simulink model "Lab_Electrical_System"  (R2018a)
settings: Solver=VariableStepAuto  StartTime=0.0  StopTime=10  RelTol=1e-3
libraries: dspsrcs4 x1
settings Model: Creator=samak-twins  LastModifiedBy=samak

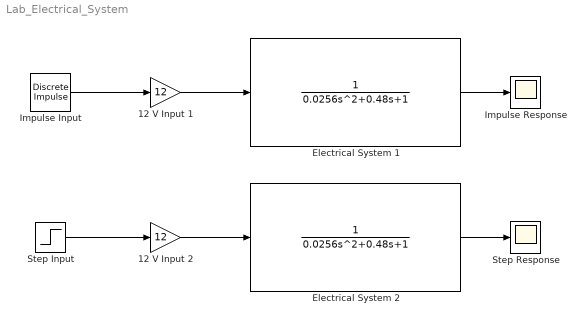
== system Lab_Electrical_System ==
  12 V Input 1 : Gain  Gain=12
  12 V Input 2 : Gain  Gain=12
  Electrical System 1 : TransferFcn  Denominator=[0.0256 0.48 1]
  Electrical System 2 : TransferFcn  Denominator=[0.0256 0.48 1]
  Impulse Input : dspsrcs4/Discrete  Impulse  Delay=0  SampleTime=1  FrameSample=1  OutputFrames=off  dataType=double  isSigned=on  wordLen=16  udDataType=sfix(16)  fracBitsMode=Best precision  numFracBits=15  OutDataTypeStr=double  LastOutDataTypeStr=double
  Impulse Response : Scope
  Step Input : Step  Time=0  SampleTime=0
  Step Response : Scope
  wires:
  Step Input/1 -> 12 V Input 2/1
  Electrical System 2/1 -> Step Response/1
  12 V Input 1/1 -> Electrical System 1/1
  12 V Input 2/1 -> Electrical System 2/1
  Impulse Input/1 -> 12 V Input 1/1
  Electrical System 1/1 -> Impulse Response/1
